simulink library "TransportDelay_lib"  (Simulink 7.2)
settings: Solver=ode45  StartTime=0.0  StopTime=10.0  RelTol=1e-3
settings Model: Creator=la1032aw  LastModifiedBy=la1032aw

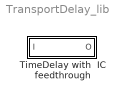
== system TransportDelay_lib ==
  TimeDelay with  IC feedthrough : Subsystem  mask{TimeDelay=10e-3}
      mask prompts: TimeDelay "Time Delay (sec)"
      mask help:
      | Implements Continuous Time Transport Delay with initial
      | outputs set to feedthrough with no delay.
      |
      |   output = input;   for t<TimeDelay
      |   output = input(t-tdelay); for t>=TimeDelay

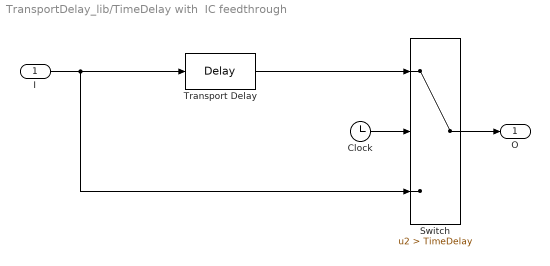
== system TransportDelay_lib/TimeDelay with  IC feedthrough ==
  I : Inport
  Clock : Clock
      settings: Decimation=10
  Switch : Switch  Criteria=u2 > Threshold  Threshold=TimeDelay  OutDataType=sfix(16)  OutScaling=2^0
  Transport Delay : TransportDelay  DelayTime=TimeDelay
      settings: AttributesFormatString=%<DelayTime>
  O : Outport
  wires:
  Transport Delay/1 -> Switch/1
  Switch/1 -> O/1
  Clock/1 -> Switch/2
  I/1 -> Switch/3, Transport Delay/1
